simulink model "S3_p4"  (R2019a)
settings: Solver=VariableStepAuto  StartTime=0.0  StopTime=10.0  RelTol=1e-3  EnableMultiTasking=on
values from neighbouring files (symbols this model uses):
  A = [0 1 0 -1;-(ks/ms) -(cs/ms) 0 cs/ms; 0 0 0 1;ks/mu cs/mu -kt/mu -(cs+ct)/mu]    [S2_P1_and_2.m]    (also in S3_P1.m; S3_P2.m; S3_P3.m; S3_P4.m)
  B = [0;1/ms;0;-1/mu]    [S2_P1_and_2.m]    (also in S3_P1.m = [0;0;-1;ct/mu]; S3_P2.m = [0 0;0 1/ms;-1 0;ct/mu -1/mu]; S3_P3.m = [0;0;-1;ct/mu]; S3_P4.m = [0 0;0 1/ms;-1 0;ct/mu -1/mu])
  C = [1 0 0 0;-(ks/ms) -(cs/ms) 0 cs/ms]    [S2_P1_and_2.m]    (also in S3_P1.m; S3_P2.m; S3_P3.m; S3_P4.m)
  D = [0;1/ms]    [S2_P1_and_2.m]    (also in S3_P1.m = [0;1]; S3_P2.m = [0 0;1 1/ms]; S3_P3.m = [0;1]; S3_P4.m = [0 0;1 1/ms])
undefined symbols (not defined in the file or in its folder): Continuous, sigbuilder_block, Time
libraries: simulink x2, ctrlSharedLib x1
settings Model: Creator=Niusha  LastModifiedBy=Sahand
settings DataIOCC: LimitDataPoints=on  ReturnWorkspaceOutputs=off
settings OptimizationCC: LifeSpan=inf
settings DebuggingCC: AllowSymbolicDim=off  SFUnexpectedBacktrackingDiag=warning  SFNoUnconditionalDefaultTransitionDiag=warning  SFExecutionAtInitializationDiag=none  ArithmeticOperatorsInVariantConditions=warning
settings ModelReferenceCC: PropagateSignalLabelsOutOfModel=off
settings SFSimCC: SimUseLocalCustomCode=off
settings RTWCC: RTWUseLocalCustomCode=off
settings CodeAppCC: StateflowObjectComments=on
settings GRTTargetCC: TargetLangStandard=C89/C90 (ANSI)
settings ConfigComp: CovMetricSettings=dw  CovHtmlReporting=on  CovSaveCumulativeToWorkspaceVar=on  CovSaveSingleToWorkspaceVar=on  CovExternalEMLEnable=off

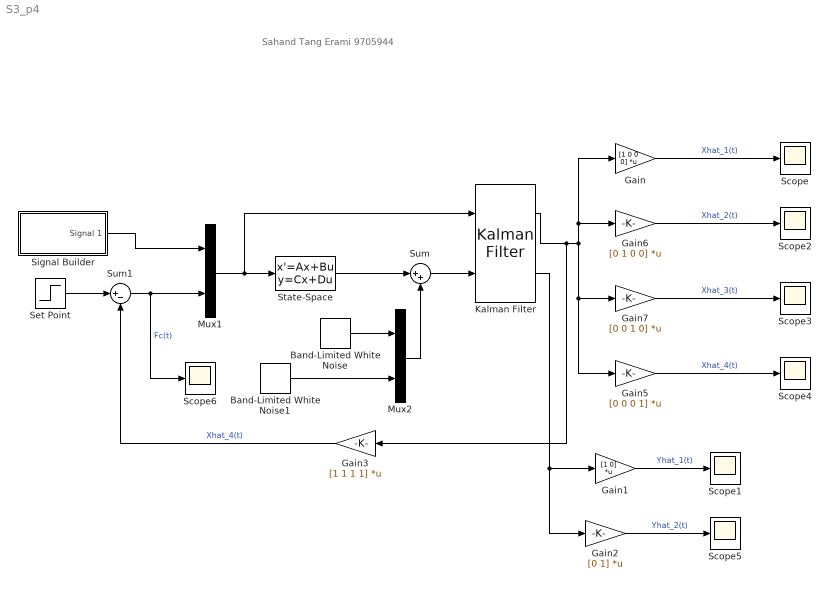
== system S3_p4 ==
  note: Sahand Tang Erami
      | 9705944
  Band-Limited White Noise : simulink/Sources/Band-Limited White Noise  Cov=.1e-6  Ts=0.1  seed=[23341]
  Band-Limited White Noise1 : simulink/Sources/Band-Limited White Noise  Cov=.1e-6  Ts=0.1  seed=[23341]
  Gain : Gain  Gain=[1 0 0 0]  Multiplication=Matrix(K*u)
  Gain1 : Gain  Gain=[1 0]  Multiplication=Matrix(K*u)
  Gain2 : Gain  Gain=[0 1]  Multiplication=Matrix(K*u)
  Gain3 : Gain  Gain=[1 1 1 1]  Multiplication=Matrix(K*u)
  Gain5 : Gain  Gain=[0 0 0 1]  Multiplication=Matrix(K*u)
  Gain6 : Gain  Gain=[0 1 0 0]  Multiplication=Matrix(K*u)
  Gain7 : Gain  Gain=[0 0 1 0]  Multiplication=Matrix(K*u)
  Kalman Filter : ctrlSharedLib/Kalman Filter  TimeDomain=Continuous-Time  UseCurrentEstimator=on  ModelSource=Individual A, B, C, D matrices  ModelSourceVariable=ss(0.95,1,1,0,1)  A=A  B=B  C=C  D=D  NumberOfStates=1  NumberOfInputs=1  NumberOfOutputs=1  InitialEstimateSource=Dialog  X0=0  P0=10  UseK=off  UseGH=off  NumberOfProcessNoiseInputs=1  G=1  TimeInvariantG=on  H=0  TimeInvariantH=on  Q=0  TimeInvariantQ=on  R=[0.01e-6 0;0 0.01e-6]  TimeInvariantR=on  N=0  TimeInvariantN=on  AddInputPort=on  AddEnablePort=off  OutputEstimatedY=on  OutputP=off  Ts=-1
      settings: SourceProductBaseCode=CT
  Mux1 : Mux  Inputs=2
  Mux2 : Mux  Inputs=2
  Scope{,1..6} (7 alike) : Scope
  Set Point : Step  Time=0  After=0  SampleTime=0
  Signal Builder : Subsystem  Tag=STV Subsys  LoadFcn=sigbuilder_block('load');  StartFcn=sigbuilder_block('start');  StopFcn=sigbuilder_block('stop');  ClipboardFcn=sigbuilder_block('clipboard');  mask(Sigbuilder block){tuvar=[0:10]}
      mask help: Simulink:masks:SigbuilderBlock_MD
      mask init:
      | if ~strcmp(get_param(bdroot(gcbh),'SimulationStatus'),'stopped') tuvar = sigbuilder_block('maskInit'); end
      settings: CopyFcn=sigbuilder_block('copy');  DeleteFcn=sigbuilder_block('delete');  ModelCloseFcn=sigbuilder_block('modelClose');  PreSaveFcn=sigbuilder_block('preSave');  PauseFcn=sigbuilder_block('pause');  ContinueFcn=sigbuilder_block('continue');  NameChangeFcn=sigbuilder_block('namechange');  OpenFcn=sigbuilder_block('open',[437.6 199.2 550.4 400 ]);  CloseFcn=sigbuilder_block('close');
      mask Display: plot(0, 0, 100, 100,[2, 2, 32, 32, 2], [68, 8, 8, 68, 68],[32, 2], [38, 38], [32, 19, 2],[53, 60, 44], [32, 17, 17, 2],[16, 16, 31, 31]);txt = getActiveGroup(gcbh);text(2, 100, txt,'verticalAlignment', 'top');
  State-Space : StateSpace  A=A  B=B  C=C  D=D  InitialCondition=[-0.001;-0.001;-0.001;-0.001]
  Sum : Sum  Inputs=|++
  Sum1 : Sum  Inputs=|+-
  wires:
  Signal Builder/1(Signal 1) -> Mux1/1
  Mux1/1 -> Kalman Filter/1, State-Space/1
  State-Space/1 -> Sum/1
  Band-Limited White Noise/1 -> Mux2/1
  Band-Limited White Noise1/1 -> Mux2/2
  Mux2/1 -> Sum/2
  Sum/1 -> Kalman Filter/2
  Gain/1 -> Scope/1  "Xhat_1(t)"
  Gain6/1 -> Scope2/1  "Xhat_2(t)"
  Gain7/1 -> Scope3/1  "Xhat_3(t)"
  Gain5/1 -> Scope4/1  "Xhat_4(t)"
  Kalman Filter/1 -> Gain6/1, Gain/1, Gain5/1, Gain7/1, Gain3/1
  Set Point/1 -> Sum1/1
  Sum1/1 -> Scope6/1, Mux1/2  "Fc(t)"
  Kalman Filter/2 -> Gain2/1, Gain1/1
  Gain1/1 -> Scope1/1  "Yhat_1(t)"
  Gain2/1 -> Scope5/1  "Yhat_2(t)"
  Gain3/1 -> Sum1/2  "Xhat_4(t)"

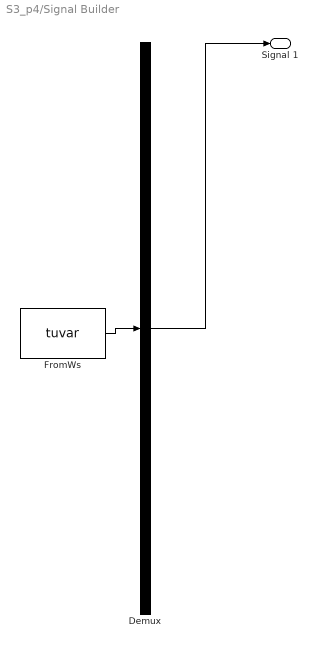
== system S3_p4/Signal Builder ==
  Demux : Demux  Tag=STV Demux  Outputs=1
  FromWs : FromWorkspace  Tag=STV FromWs  VariableName=tuvar  SampleTime=0
      SigBuilderData=|
      | common.afterFinalStr = 'Extrapolate'
      | common.sampleTime = 0
      | dataSet.timeRange = [0 10]
      | dataSet.name = 'Group 1'
      | sbobj.Groups.Name = 'Group 1'
      | sbobj.Groups.Signals.Name = 'Signal 1'
      | sbobj.Groups.Signals.XData = [0 0.02 0.02 10]
      | sbobj.Groups.Signals.YData = [0.1 0.1 0 0]
  Signal 1 : Outport  Tag=STV Outport
  wires:
  Demux/1 -> Signal 1/1
  FromWs/1 -> Demux/1
